simulink model "Small_signal_model_DCDC"  (R2021a)
settings: Solver=VariableStepAuto  StartTime=0.0  StopTime=10.0  RelTol=1e-3
settings Model: Creator=prizm  LastModifiedBy=prizm

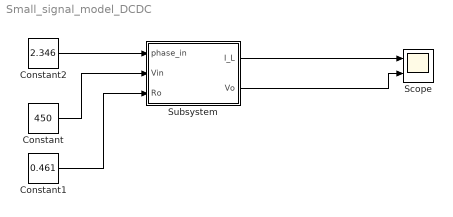
== system Small_signal_model_DCDC ==
  Constant : Constant  Value=450
  Constant1 : Constant  Value=0.461
  Constant2 : Constant  Value=2.346
  Scope : Scope  NumInputPorts=2
  Subsystem : Subsystem  mask{Lo=10e-6, Co=1e-3, n=0.143}
      mask prompts: Lo "Output Inductor"; Co "Output Capacitor"; n "Transformer Turns ratio"
  wires:
  Constant/1 -> Subsystem/2(Vin)
  Constant1/1 -> Subsystem/3(Ro)
  Constant2/1 -> Subsystem/1(phase_in)
  Subsystem/1(I_L) -> Scope/1
  Subsystem/2(Vo) -> Scope/2

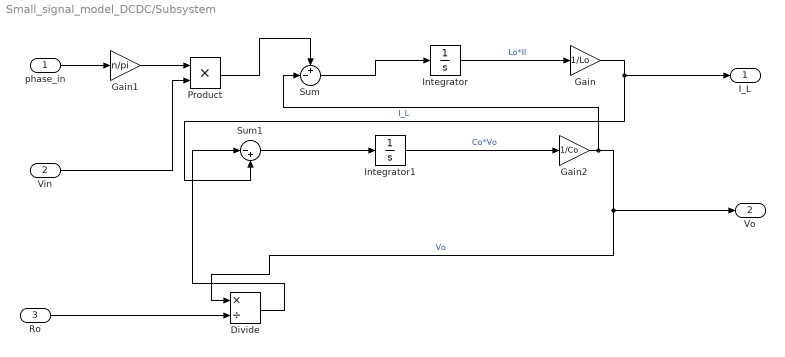
== system Small_signal_model_DCDC/Subsystem ==
  phase_in : Inport
  Vin : Inport  Port=2
  Ro : Inport  Port=3
  Divide : Product  Inputs=*/
  Gain : Gain  Gain=1/Lo
  Gain1 : Gain  Gain=n/pi
  Gain2 : Gain  Gain=1/Co
  Integrator : Integrator
  Integrator1 : Integrator
  Product : Product
  Sum : Sum  Inputs=+-|
  Sum1 : Sum  Inputs=|-+
  I_L : Outport
  Vo : Outport  Port=2
  wires:
  Gain1/1 -> Product/1
  Product/1 -> Sum/1
  Divide/1 -> Sum1/1
  Integrator1/1 -> Gain2/1  "Co*Vo"
  Gain2/1 -> Vo/1, Divide/1, Sum/2  "Vo"
  phase_in/1 -> Gain1/1
  Gain/1 -> I_L/1, Sum1/2  "I_L"
  Integrator/1 -> Gain/1  "Lo*Il"
  Sum1/1 -> Integrator1/1
  Sum/1 -> Integrator/1
  Vin/1 -> Product/2
  Ro/1 -> Divide/2
